simulink model "Switch_pulse_for_single_phase_inverter"  (R2019a)
settings: Solver=VariableStepAuto  StartTime=0.0  StopTime=3/60  RelTol=1e-3
libraries: powerlib x1
settings Model: Creator=Ram Baskar  LastModifiedBy=Ram Baskar

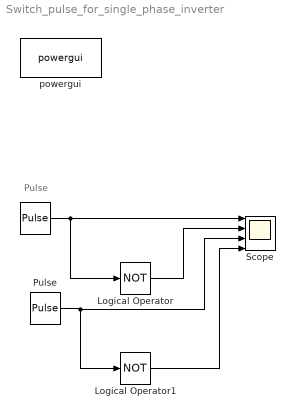
== system Switch_pulse_for_single_phase_inverter ==
  note: Pulse
  " " : DiscretePulseGenerator  PulseType=Time based  Period=16.66667e-3  PulseWidth=50  PhaseDelay=-1.38889e-3
  Logical Operator : Logic  Operator=NOT  AllPortsSameDT=off  OutDataTypeStr=boolean
  Logical Operator1 : Logic  Operator=NOT  AllPortsSameDT=off  OutDataTypeStr=boolean
  Pulse : DiscretePulseGenerator  PulseType=Time based  Period=16.66667e-3  PulseWidth=50  PhaseDelay=-6.94444e-3
  Scope : Scope  NumInputPorts=4
  powergui : powerlib/powergui  Priority=1  SimulationMode=Continuous  SampleTime=50e-6  frequency=60  Iterations=50  frequencyindice=60  Pbase=100e6  ErrMax=1e-4  UnitsV=kV  UnitsW=MW  buscounter=0  FunctionMessages=off  echomessages=off  EnableUseOfTLC=off  CurrentSourceSwitches=off  DisableSnubberDevices=off  DisableRonSwitches=off  DisableVfSwitches=off  DisplayEquations=off  AutomaticDiscreteSolvers=off  SolverType=Tustin/Backward Euler (TBE)  Interpol=off  ExternalGateDelay=off  methode=off  Ts=100  x0status=blocks  SPID=on  SwTol=0  HookPort=off  NonlinearTolerance=0  nMaxIteration=15  ContinueOnMaxIteration=off  RestoreLinks=warning  ResistiveCurrentMeasurement=off  Frange=[0:2:500]  Ylog=off  Xlog=on  ShowGrid=off  save=off  variable=ZData  structure=0  ZoomFFT=off  StartTime=0.0  cycles=1  DisplayStyle=1  fundamental=60  FreqAxis=off  MaxFrequency=1000  frequencyindicesteady=1  RmsSteady=1  display=off
      settings: SourceProductName=Simscape Electrical
  wires:
  " "/1 -> Logical Operator/1, Scope/1
  Logical Operator/1 -> Scope/2
  Logical Operator1/1 -> Scope/4
  Pulse/1 -> Logical Operator1/1, Scope/3
